simulink model "Well2_FluidLoop"  (R2019b)
settings: Solver=ode23t  StartTime=0.0  StopTime=40  RelTol=1e-3
PreLoadFcn:
  | init_press=900;
  | trapped_air=0.0007;
  | SPM=30;
  | Choke=0.25;
libraries: sh_lib x16, fl_lib x11, nesl_utility x8, simulink x3
settings Model: Creator=charl  LastModifiedBy=charl
settings SFSimCC: CustomCodeUndefinedFunction=UseInterfaceOnly

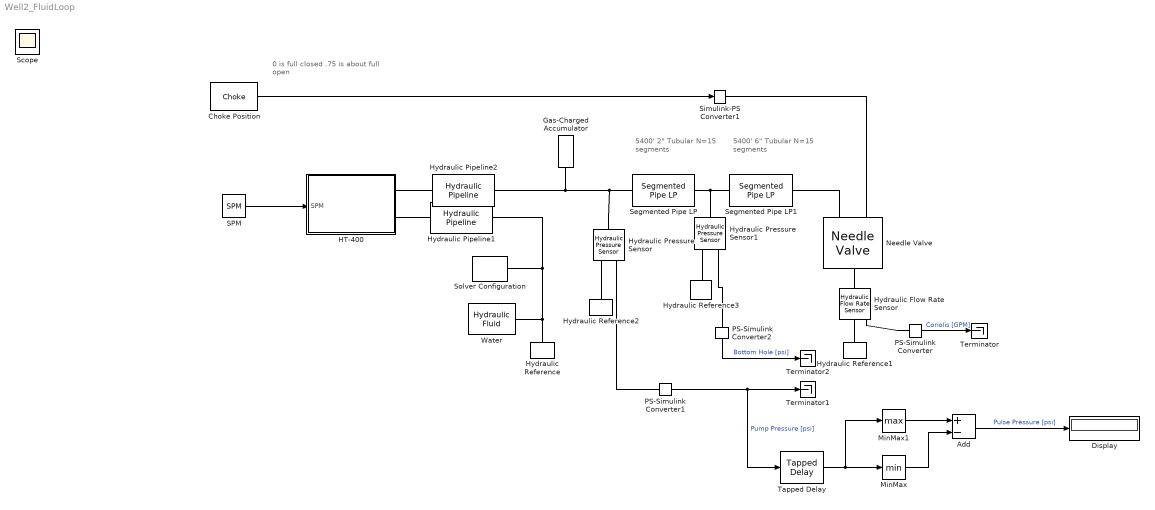
== system Well2_FluidLoop ==
  note: 0 is full closed
      | .75 is about full open
  note: 5400' 2" Tubular
      | N=15 segments
  note: 5400' 6" Tubular
      | N=15 segments
  Add : Sum  Inputs=+-
  Choke Position : Constant  Value=Choke
  Display : Display
  Gas-Charged Accumulator : sh_lib/Accumulators/Gas-Charged Accumulator  capacity=10 gal  dead_volume=1 gal  pr_preload=init_press psi  k_sh=1.4  stiff_coeff=1e10 Pa/m^3  penetr_coeff=1e10 s*Pa/m^6  flow_rate_specify=off  flow_rate_priority=None  flow_rate=0.005 m^3/s  flow_rate_nominal_specify=off  flow_rate_nominal_unit=m^3/s  flow_rate_nominal_value=1  liquid_volume_specify=off  liquid_volume_priority=High  liquid_volume=100 gal  liquid_volume_nominal_specify=off  liquid_volume_nominal_unit=m^3  liquid_volume_nominal_value=1  liquid_pressure_specify=off  liquid_pressure_priority=None  liquid_pressure=1.01325e+5 Pa  liquid_pressure_nominal_specify=off  liquid_pressure_nominal_unit=Pa  liquid_pressure_nominal_value=1
      settings: SourceProductName=Simscape Fluids  SourceProductBaseCode=SH  InternalSimscapePortConfiguration="{\"Bottom\":[],\"Left\":[],\"Right\":[{\"id\":\"A\",\"label\":\"A\",\"type\":\"foundation.hydraulic.hydraulic\"}],\"Top\":[]}"
  HT-400 : Subsystem
  Hydraulic Flow Rate Sensor : fl_lib/Hydraulic/Hydraulic Sensors/Hydraulic Flow Rate Sensor
      settings: SourceProductName=Simscape
  Hydraulic Pipeline1 : sh_lib/Pipelines/Hydraulic Pipeline  cs_type=1  d_in=4 in  area=1e-4 m^2  D_h=1.12e-2 m  s_factor=64  length=20 ft  length_ad=1 ft  roughness=15e-6 m  Re_lam=2000  Re_turb=4000  wall_type=1  pr_r_coef=2e-12 m/Pa  time_const=0.01 s  k_sh=1.4  initial_pressure=0 Pa
      settings: SourceProductName=Simscape Fluids  SourceProductBaseCode=SH  InternalSimscapePortConfiguration="{\"Bottom\":[],\"Left\":[{\"id\":\"A\",\"label\":\"A\",\"type\":\"foundation.hydraulic.hydraulic\"}],\"Right\":[{\"id\":\"B\",\"label\":\"B\",\"type\":\"foundation.hydraulic.hydraulic\"}],\"Top\":[]}"
  Hydraulic Pipeline2 : sh_lib/Pipelines/Hydraulic Pipeline  cs_type=1  d_in=4 in  area=1e-4 m^2  D_h=1.12e-2 m  s_factor=64  length=10 ft  length_ad=1 ft  roughness=15e-6 m  Re_lam=2000  Re_turb=4000  wall_type=1  pr_r_coef=2e-12 m/Pa  time_const=0.01 s  k_sh=1.4  initial_pressure=0 Pa
      settings: SourceProductName=Simscape Fluids  SourceProductBaseCode=SH  InternalSimscapePortConfiguration="{\"Bottom\":[],\"Left\":[{\"id\":\"A\",\"label\":\"A\",\"type\":\"foundation.hydraulic.hydraulic\"}],\"Right\":[{\"id\":\"B\",\"label\":\"B\",\"type\":\"foundation.hydraulic.hydraulic\"}],\"Top\":[]}"
  Hydraulic Pressure Sensor : fl_lib/Hydraulic/Hydraulic Sensors/Hydraulic Pressure Sensor
      settings: SourceProductName=Simscape
  Hydraulic Pressure Sensor1 : fl_lib/Hydraulic/Hydraulic Sensors/Hydraulic Pressure Sensor
      settings: SourceProductName=Simscape
  Hydraulic Reference{,1..3} (4 alike) : fl_lib/Hydraulic/Hydraulic Elements/Hydraulic Reference
      settings: SourceProductName=Simscape
  MinMax : MinMax
  MinMax1 : MinMax  Function=max
  Needle Valve : sh_lib/Valves/Flow Control Valves/Needle Valve  d_orif=2 in  cone_angle=90 deg  x_0=.25 in  C_d=0.65  A_leak=1e-12 m^2  lam_spec=1  B_lam=0.999  Re_cr=10
      settings: SourceProductName=Simscape Fluids  SourceProductBaseCode=SH  InternalSimscapePortConfiguration="{\"Bottom\":[],\"Left\":[{\"id\":\"S\",\"label\":\"S\",\"type\":\"input\"},{\"id\":\"A\",\"label\":\"A\",\"type\":\"foundation.hydraulic.hydraulic\"}],\"Right\":[{\"id\":\"B\",\"label\":\"B\",\"type\":\"foundation.hydraulic.hydraulic\"}],\"Top\":[]}"
  PS-Simulink Converter : nesl_utility/PS-Simulink Converter  PhysicalDomain=network_engine_domain  SubClassName=ps_output  LeftPortType=input  RightPortType=output  PseudoPeriodic=off  Frequencies=[]  Unit=gpm  AffineConversion=off
  PS-Simulink Converter1 : nesl_utility/PS-Simulink Converter  PhysicalDomain=network_engine_domain  SubClassName=ps_output  LeftPortType=input  RightPortType=output  PseudoPeriodic=off  Frequencies=[]  Unit=psi  AffineConversion=off
  PS-Simulink Converter2 : nesl_utility/PS-Simulink Converter  PhysicalDomain=network_engine_domain  SubClassName=ps_output  LeftPortType=input  RightPortType=output  PseudoPeriodic=off  Frequencies=[]  Unit=psi  AffineConversion=off
  SPM : Constant  Value=SPM
  Segmented Pipe LP : sh_lib/Low-Pressure Blocks/Segmented Pipe LP  d_in=2 in  length=5400 ft  segm_num=round(4*(5500)/(pi()*4672)*10)  length_ad=1 m  roughness=1.5e-5 m  Re_lam=2e+3  Re_turb=4e+3  elevation_A=5400 ft  elevation_B=0 ft  g=9.806649999999999 m/s^2  wall_type=1  pr_r_coef=2e-10 m/Pa  time_const=0.008 s  k_sh=1.4  p0_vec=init_press psi  q0=0 m^3/s
      settings: SourceProductName=Simscape Fluids  SourceProductBaseCode=SH  InternalSimscapePortConfiguration="{\"Bottom\":[],\"Left\":[{\"id\":\"A\",\"label\":\"A\",\"type\":\"foundation.hydraulic.hydraulic\"}],\"Right\":[{\"id\":\"B\",\"label\":\"B\",\"type\":\"foundation.hydraulic.hydraulic\"}],\"Top\":[]}"
  Segmented Pipe LP1 : sh_lib/Low-Pressure Blocks/Segmented Pipe LP  d_in=6 in  length=5400 ft  segm_num=round(4*(5500)/(pi()*4672)*10)  length_ad=1 m  roughness=1.5e-5 m  Re_lam=2e+3  Re_turb=4e+3  elevation_A=0 ft  elevation_B=5400 ft  g=9.806649999999999 m/s^2  wall_type=1  pr_r_coef=2e-10 m/Pa  time_const=0.008 s  k_sh=1.4  p0_vec=init_press psi  q0=0 m^3/s
      settings: SourceProductName=Simscape Fluids  SourceProductBaseCode=SH  InternalSimscapePortConfiguration="{\"Bottom\":[],\"Left\":[{\"id\":\"A\",\"label\":\"A\",\"type\":\"foundation.hydraulic.hydraulic\"}],\"Right\":[{\"id\":\"B\",\"label\":\"B\",\"type\":\"foundation.hydraulic.hydraulic\"}],\"Top\":[]}"
  Simulink-PS Converter1 : nesl_utility/Simulink-PS Converter  PhysicalDomain=network_engine_domain  SubClassName=ps_input  LeftPortType=input  RightPortType=output  PseudoPeriodic=off  Frequencies=[]  NoiseDistribution=none  NoiseParameters=[]  Unit=in  AffineConversion=off  FilteringAndDerivatives=provide  SimscapeFilterOrder=1  InputFilterTimeConstant=0.001  UdotUserProvided=0
  Solver Configuration : nesl_utility/Solver Configuration  PhysicalDomain=network_engine_domain  SubClassName=solver  LeftPortType=input  RightPortType=generic  Tones=[]  Harmonics=[]  SimulateNoise=off  Profile=off  UseLocalSampling=off  EnableSwitchedLinearOptims=on  FrequencyDomain=off  UseCCode=off  RelTol=0.001  AbsTol=1e-06  MinStep=1e-09  ToWorkspace=off  RevertToSquareIcSolve=off  NumHomotopyIterations=100  PhasorMode=off  PhasorModeNumHarmonics=1  DoDC=off  ResidualTolerance=1e-09  UseLocalSolver=off  LocalSolverChoice=NE_BACKWARD_EULER_ADVANCER  LocalSolverSampleTime=0.001  DoFixedCost=off  MaxNonlinIter=3  MaxModeIter=2  LinearAlgebra=auto  EquationFormulation=NE_TIME_EF  DelaysMemoryBudget=1024  AutomaticFiltering=on  FilteringTimeConstant=0.001  PartitionStorageMethod=AS_NEEDED  PartitionMemoryBudget=1024  PartitionMethod=ROBUST
  Tapped Delay : simulink/Discrete/Tapped Delay  vinit=0  samptime=-1  NumDelays=1E4  DelayOrder=Oldest  includeCurrent=off
  Terminator : Terminator
  Terminator1 : Terminator
  Terminator2 : Terminator
  Water : sh_lib/Hydraulic Utilities/Hydraulic Fluid  DataSource=1  SelFluid=24  SysTemp=22  TrapAir=0.007  ViscDerFactor=1  range_error=2
      settings: SourceProductName=Simscape Fluids
  Scope : Scope
  wires:
  Choke Position/1 -> Simulink-PS Converter1/1
  PS-Simulink Converter/1 -> Terminator/1  "Coriolis [GPM]"
  PS-Simulink Converter1/1 -> Tapped Delay/1, Terminator1/1  "Pump Pressure [psi]"
  SPM/1 -> HT-400/1(SPM)
  Tapped Delay/1 -> MinMax1/1, MinMax/1
  MinMax1/1 -> Add/1
  MinMax/1 -> Add/2
  Add/1 -> Display/1  "Pulse Pressure [psi]"
  PS-Simulink Converter2/1 -> Terminator2/1  "Bottom Hole [psi]"
  connections:
  Hydraulic Reference/LConn1 -- Hydraulic Pipeline1/RConn1 -- Solver Configuration/RConn1 -- Water/RConn1
  Simulink-PS Converter1/RConn1 -- Needle Valve/LConn1
  Hydraulic Flow Rate Sensor/LConn1 -- Needle Valve/RConn1
  Hydraulic Flow Rate Sensor/RConn2 -- Hydraulic Reference1/LConn1
  PS-Simulink Converter/LConn1 -- Hydraulic Flow Rate Sensor/RConn1
  Hydraulic Reference2/LConn1 -- Hydraulic Pressure Sensor/RConn1
  Hydraulic Pressure Sensor/RConn2 -- PS-Simulink Converter1/LConn1
  Hydraulic Pipeline2/RConn1 -- Segmented Pipe LP/LConn1 -- Hydraulic Pressure Sensor/LConn1 -- Gas-Charged Accumulator/RConn1
  HT-400/RConn1 -- Hydraulic Pipeline2/LConn1
  Hydraulic Pipeline1/LConn1 -- HT-400/RConn2
  Segmented Pipe LP1/LConn1 -- Hydraulic Pressure Sensor1/LConn1 -- Segmented Pipe LP/RConn1
  Segmented Pipe LP1/RConn1 -- Needle Valve/LConn2
  Hydraulic Pressure Sensor1/RConn2 -- PS-Simulink Converter2/LConn1
  Hydraulic Reference3/LConn1 -- Hydraulic Pressure Sensor1/RConn1

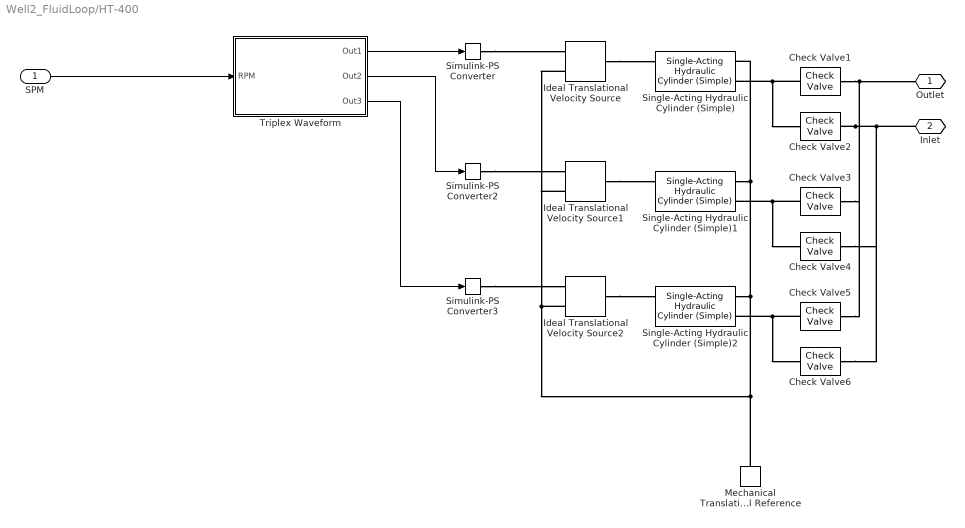
== system Well2_FluidLoop/HT-400 ==
  SPM : Inport
  Check Valve{1..6} (6 alike) : sh_lib/Valves/Directional Valves/Check Valve  area_max=(1)*pi() in^2  pres_crack=0.3e5 Pa  pres_max=1.2e5 Pa  C_d=0.7  A_leak=1e-12 m^2  lam_spec=1  B_lam=0.999  Re_cr=12  dynamic=0  tau=0.1 s  area_init=1e-12 m^2
      settings: SourceProductName=Simscape Fluids  SourceProductBaseCode=SH  InternalSimscapePortConfiguration="{\"Bottom\":[],\"Left\":[{\"id\":\"A\",\"label\":\"A\",\"type\":\"foundation.hydraulic.hydraulic\"}],\"Right\":[{\"id\":\"B\",\"label\":\"B\",\"type\":\"foundation.hydraulic.hydraulic\"}],\"Top\":[]}"
  Ideal Translational Velocity Source : fl_lib/Mechanical/Mechanical Sources/Ideal Translational Velocity Source
  Ideal Translational Velocity Source1 : fl_lib/Mechanical/Mechanical Sources/Ideal Translational Velocity Source
  Ideal Translational Velocity Source2 : fl_lib/Mechanical/Mechanical Sources/Ideal Translational Velocity Source
  Mechanical Translational Reference : fl_lib/Mechanical/Translational Elements/Mechanical Translational Reference
  Simulink-PS Converter : nesl_utility/Simulink-PS Converter  PhysicalDomain=network_engine_domain  SubClassName=ps_input  LeftPortType=input  RightPortType=output  PseudoPeriodic=off  Frequencies=[]  NoiseDistribution=none  NoiseParameters=[]  Unit=in/s  AffineConversion=off  FilteringAndDerivatives=provide  SimscapeFilterOrder=1  InputFilterTimeConstant=0.001  UdotUserProvided=0
  Simulink-PS Converter2 : nesl_utility/Simulink-PS Converter  PhysicalDomain=network_engine_domain  SubClassName=ps_input  LeftPortType=input  RightPortType=output  PseudoPeriodic=off  Frequencies=[]  NoiseDistribution=none  NoiseParameters=[]  Unit=in/s  AffineConversion=off  FilteringAndDerivatives=provide  SimscapeFilterOrder=1  InputFilterTimeConstant=0.001  UdotUserProvided=0
  Simulink-PS Converter3 : nesl_utility/Simulink-PS Converter  PhysicalDomain=network_engine_domain  SubClassName=ps_input  LeftPortType=input  RightPortType=output  PseudoPeriodic=off  Frequencies=[]  NoiseDistribution=none  NoiseParameters=[]  Unit=in/s  AffineConversion=off  FilteringAndDerivatives=provide  SimscapeFilterOrder=1  InputFilterTimeConstant=0.001  UdotUserProvided=0
  Single-Acting Hydraulic Cylinder (Simple) : sh_lib/Hydraulic Cylinders/Single-Acting Hydraulic Cylinder (Simple)  area=(3^2)*pi() in^2  stroke=24 in  init_pos=12 in  penetr_coeff=1e12 s*N/m^2  or=1
      settings: SourceProductName=Simscape Fluids  SourceProductBaseCode=SH  InternalSimscapePortConfiguration="{\"Bottom\":[],\"Left\":[{\"id\":\"C\",\"label\":\"C\",\"type\":\"foundation.mechanical.translational.translational\"},{\"id\":\"A\",\"label\":\"A\",\"type\":\"foundation.hydraulic.hydraulic\"}],\"Right\":[{\"id\":\"R\",\"label\":\"R\",\"type\":\"foundation.mechanical.translational.translational\"},{\"id\":\"P\",\"label\":\"P\",\"type\":\"output\"}],\"Top\":[]}"
  Single-Acting Hydraulic Cylinder (Simple)1 : sh_lib/Hydraulic Cylinders/Single-Acting Hydraulic Cylinder (Simple)  area=(3^2)*pi() in^2  stroke=24 in  init_pos=12+12*sin(2*pi()/3) in  penetr_coeff=1e12 s*N/m^2  or=1
      settings: SourceProductName=Simscape Fluids  SourceProductBaseCode=SH  InternalSimscapePortConfiguration="{\"Bottom\":[],\"Left\":[{\"id\":\"C\",\"label\":\"C\",\"type\":\"foundation.mechanical.translational.translational\"},{\"id\":\"A\",\"label\":\"A\",\"type\":\"foundation.hydraulic.hydraulic\"}],\"Right\":[{\"id\":\"R\",\"label\":\"R\",\"type\":\"foundation.mechanical.translational.translational\"},{\"id\":\"P\",\"label\":\"P\",\"type\":\"output\"}],\"Top\":[]}"
  Single-Acting Hydraulic Cylinder (Simple)2 : sh_lib/Hydraulic Cylinders/Single-Acting Hydraulic Cylinder (Simple)  area=(3^2)*pi() in^2  stroke=24 in  init_pos=12+12*sin(4*pi()/3) in  penetr_coeff=1e12 s*N/m^2  or=1
      settings: SourceProductName=Simscape Fluids  SourceProductBaseCode=SH  InternalSimscapePortConfiguration="{\"Bottom\":[],\"Left\":[{\"id\":\"C\",\"label\":\"C\",\"type\":\"foundation.mechanical.translational.translational\"},{\"id\":\"A\",\"label\":\"A\",\"type\":\"foundation.hydraulic.hydraulic\"}],\"Right\":[{\"id\":\"R\",\"label\":\"R\",\"type\":\"foundation.mechanical.translational.translational\"},{\"id\":\"P\",\"label\":\"P\",\"type\":\"output\"}],\"Top\":[]}"
  Triplex Waveform : Subsystem
  Outlet : PMIOPort  Side=Right
  Inlet : PMIOPort  Port=2  Side=Right
  wires:
  Triplex Waveform/3(Out3) -> Simulink-PS Converter3/1
  SPM/1 -> Triplex Waveform/1(RPM)
  Triplex Waveform/1(Out1) -> Simulink-PS Converter/1
  Triplex Waveform/2(Out2) -> Simulink-PS Converter2/1
  connections:
  Check Valve1/RConn1 -- Outlet/RConn1 -- Check Valve5/RConn1 -- Check Valve3/RConn1
  Simulink-PS Converter3/RConn1 -- Ideal Translational Velocity Source2/RConn1
  Simulink-PS Converter2/RConn1 -- Ideal Translational Velocity Source1/RConn1
  Mechanical Translational Reference/LConn1 -- Ideal Translational Velocity Source/RConn2 -- Ideal Translational Velocity Source1/RConn2 -- Ideal Translational Velocity Source2/RConn2 -- Single-Acting Hydraulic Cylinder (Simple)2/LConn1 -- Single-Acting Hydraulic Cylinder (Simple)/LConn1 -- Single-Acting Hydraulic Cylinder (Simple)1/LConn1
  Check Valve3/LConn1 -- Check Valve4/RConn1 -- Single-Acting Hydraulic Cylinder (Simple)1/LConn2
  Ideal Translational Velocity Source2/LConn1 -- Single-Acting Hydraulic Cylinder (Simple)2/RConn1
  Check Valve5/LConn1 -- Check Valve6/RConn1 -- Single-Acting Hydraulic Cylinder (Simple)2/LConn2
  Ideal Translational Velocity Source1/LConn1 -- Single-Acting Hydraulic Cylinder (Simple)1/RConn1
  Check Valve1/LConn1 -- Check Valve2/RConn1 -- Single-Acting Hydraulic Cylinder (Simple)/LConn2
  Check Valve2/LConn1 -- Inlet/RConn1 -- Check Valve6/LConn1 -- Check Valve4/LConn1
  Simulink-PS Converter/RConn1 -- Ideal Translational Velocity Source/RConn1
  Ideal Translational Velocity Source/LConn1 -- Single-Acting Hydraulic Cylinder (Simple)/RConn1

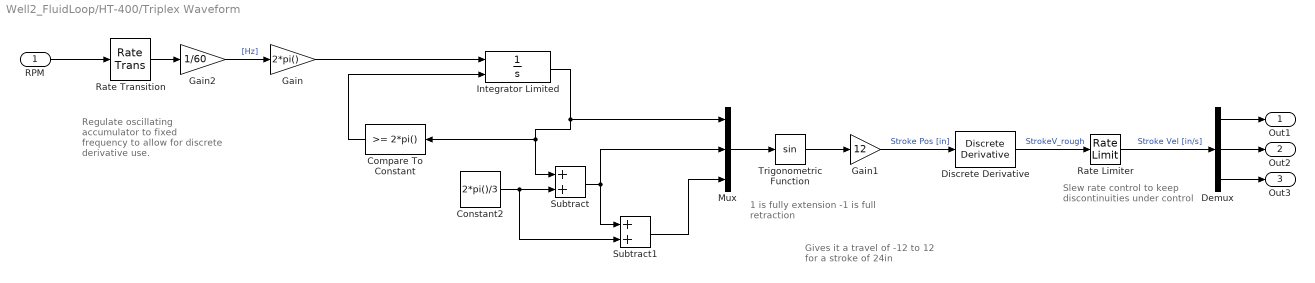
== system Well2_FluidLoop/HT-400/Triplex Waveform ==
  note: Slew rate control to keep discontinuities under control
  note: Regulate oscillating accumulator to fixed frequency to allow for discrete derivative use.
  note: Gives it a travel of -12 to 12
      | for a stroke of 24in
  note: 1 is fully extension
      | -1 is full retraction
  RPM : Inport
  Compare To Constant : simulink/Logic and Bit Operations/Compare To Constant  relop=>=  const=2*pi()  OutDataTypeStr=boolean
  Constant2 : Constant  Value=2*pi()/3
  Demux : Demux  Outputs=3
  Discrete Derivative : simulink/Discrete/Discrete Derivative  gainval=1.0  ICPrevScaledInput=0.0  OutMin=[]  OutMax=[]  OutDataType=fixdt(1, 16)  OutScaling=2^-10  DoSatur=off
  Gain : Gain  Gain=2*pi()
  Gain1 : Gain  Gain=12
  Gain2 : Gain  Gain=1/60
  Integrator Limited : Integrator  ExternalReset=rising  InitialCondition=1E-6  LimitOutput=on  UpperSaturationLimit=2*pi()  LowerSaturationLimit=0
  Mux : Mux  Inputs=3
  Rate Limiter : RateLimiter  RisingSlewLimit=100  FallingSlewLimit=-100  SampleTimeMode=inherited
  Rate Transition : RateTransition  OutPortSampleTime=.005
  Subtract : Sum
  Subtract1 : Sum
  Trigonometric Function : Trigonometry
  Out1 : Outport  VectorParamsAs1DForOutWhenUnconnected=off
  Out2 : Outport  Port=2  VectorParamsAs1DForOutWhenUnconnected=off
  Out3 : Outport  Port=3  VectorParamsAs1DForOutWhenUnconnected=off
  wires:
  Gain/1 -> Integrator Limited/1
  Compare To Constant/1 -> Integrator Limited/2
  Constant2/1 -> Subtract1/2, Subtract/2
  Subtract/1 -> Subtract1/1, Mux/2
  RPM/1 -> Rate Transition/1
  Demux/1 -> Out1/1
  Demux/2 -> Out2/1
  Demux/3 -> Out3/1
  Subtract1/1 -> Mux/3
  Mux/1 -> Trigonometric Function/1
  Gain1/1 -> Discrete Derivative/1  "Stroke Pos [in]"
  Trigonometric Function/1 -> Gain1/1
  Gain2/1 -> Gain/1  "[Hz]"
  Discrete Derivative/1 -> Rate Limiter/1  "StrokeV_rough"
  Integrator Limited/1 -> Mux/1, Compare To Constant/1, Subtract/1
  Rate Transition/1 -> Gain2/1
  Rate Limiter/1 -> Demux/1  "Stroke Vel [in/s]"
